simulink model "Now_create_a_Simulink_subsystem_which_takes_ut"  (R2021a)
settings: Solver=VariableStepAuto  StartTime=0.0  StopTime=10.0  RelTol=1e-3
libraries: dsparch4 x2, dspsigops x2, commsynccomp2 x2, simulink x2
settings Model: Creator=Fatiha  LastModifiedBy=Fatiha

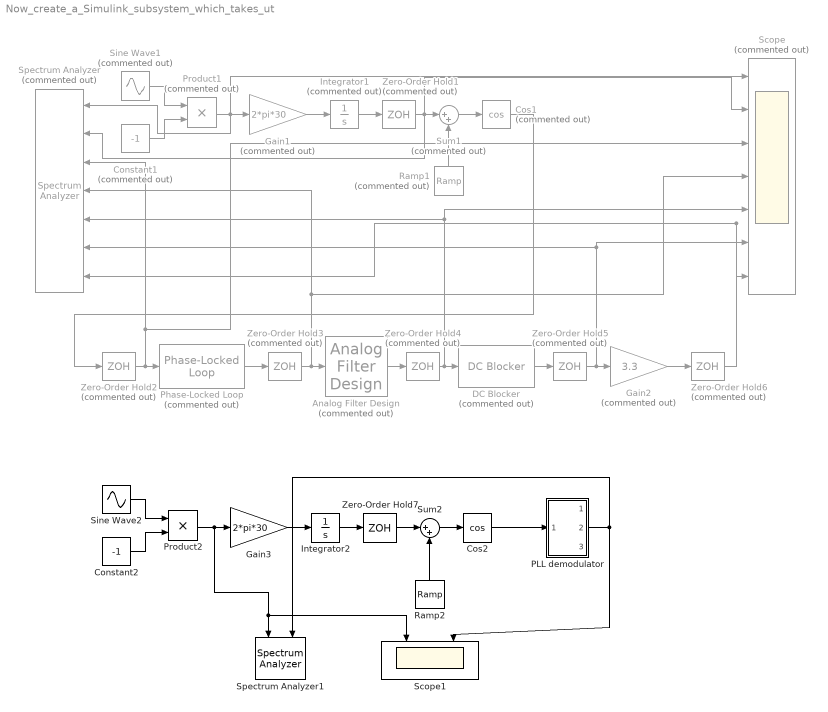
== system Now_create_a_Simulink_subsystem_which_takes_ut ==
  Analog Filter Design : dsparch4/Analog Filter Design  Commented=on  method=Butterworth  filttype=Lowpass  N=8  Wlo=2*pi*200  Whi=80  Rp=2  Rs=40
  Constant1 : Constant  Commented=on  Value=-1  SampleTime=0.00001
  Constant2 : Constant  Value=-1  SampleTime=0.00001
  Cos1 : Trigonometry  Commented=on  Operator=cos  OutputSignalType=real
  Cos2 : Trigonometry  Operator=cos  OutputSignalType=real
  DC Blocker : dspsigops/DC Blocker  Commented=on  Algorithm=IIR  NormalizedBandwidth=0.001  Length=8  Order=6  SimulateUsing=Code generation
      settings: SourceProductBaseCode=DS
  Gain1 : Gain  Commented=on  Gain=2*pi*30
  Gain2 : Gain  Commented=on  Gain=3.3
  Gain3 : Gain  Gain=2*pi*30
  Integrator1 : Integrator  Commented=on
  Integrator2 : Integrator
  PLL demodulator : Subsystem
  Phase-Locked Loop : commsynccomp2/Phase-Locked Loop  Commented=on  Fn="[3.0002  0  40002]"  Fd="[1   67.46   2270.9   40002]"  Kvco=1  Fc=200  Ph=0  Ac=1
      settings: SourceProductBaseCode=CM
  Product1 : Product  Commented=on
  Product2 : Product
  Ramp1 : simulink/Sources/Ramp  Commented=on  slope=2*pi*200  start=0  InitialOutput=0
  Ramp2 : simulink/Sources/Ramp  slope=2*pi*200  start=0  InitialOutput=0
  Scope : Scope  Commented=on  NumInputPorts=7
  Scope1 : Scope  NumInputPorts=2
  Sine Wave1 : Sin  Commented=on  Frequency=2*pi*50  SampleTime=0.00001
  Sine Wave2 : Sin  Frequency=2*pi*50  SampleTime=0.00001
  Spectrum Analyzer : SpectrumAnalyzer  Commented=on  NumInputPorts=7
  Spectrum Analyzer1 : SpectrumAnalyzer  NumInputPorts=2
  Sum1 : Sum  Commented=on  Inputs=|++
  Sum2 : Sum  Inputs=|++
  Zero-Order Hold{1..6} (6 alike) : ZeroOrderHold  Commented=on  SampleTime=0.00001
  Zero-Order Hold7 : ZeroOrderHold  SampleTime=0.00001
  wires:
  Gain1/1 -> Integrator1/1
  Sine Wave1/1 -> Product1/1
  Sum1/1 -> Cos1/1
  Constant1/1 -> Product1/2
  Product1/1 -> Spectrum Analyzer/1, Scope/1, Gain1/1
  Ramp1/1 -> Sum1/2
  Zero-Order Hold4/1 -> Spectrum Analyzer/5, Scope/5, DC Blocker/1
  Integrator1/1 -> Zero-Order Hold1/1
  Zero-Order Hold1/1 -> Spectrum Analyzer/2, Scope/2, Sum1/1
  Cos1/1 -> Zero-Order Hold2/1
  Zero-Order Hold2/1 -> Spectrum Analyzer/3, Scope/3, Phase-Locked Loop/1
  Phase-Locked Loop/2 -> Zero-Order Hold3/1
  Zero-Order Hold3/1 -> Spectrum Analyzer/4, Scope/4, Analog Filter Design/1
  Analog Filter Design/1 -> Zero-Order Hold4/1
  DC Blocker/1 -> Zero-Order Hold5/1
  Zero-Order Hold5/1 -> Scope/6, Spectrum Analyzer/6, Gain2/1
  Gain2/1 -> Zero-Order Hold6/1
  Zero-Order Hold6/1 -> Scope/7, Spectrum Analyzer/7
  Ramp2/1 -> Sum2/2
  Zero-Order Hold7/1 -> Sum2/1
  Integrator2/1 -> Zero-Order Hold7/1
  Product2/1 -> Scope1/1, Spectrum Analyzer1/1, Gain3/1
  Sum2/1 -> Cos2/1
  Constant2/1 -> Product2/2
  Gain3/1 -> Integrator2/1
  Sine Wave2/1 -> Product2/1
  Cos2/1 -> PLL demodulator/1(In1)
  PLL demodulator/2(Out2) -> Scope1/2, Spectrum Analyzer1/2

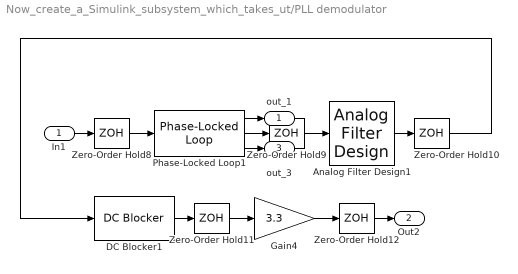
== system Now_create_a_Simulink_subsystem_which_takes_ut/PLL demodulator ==
  In1 : Inport
  Analog Filter Design1 : dsparch4/Analog Filter Design  method=Butterworth  filttype=Lowpass  N=8  Wlo=2*pi*200  Whi=80  Rp=2  Rs=40
  DC Blocker1 : dspsigops/DC Blocker  Algorithm=IIR  NormalizedBandwidth=0.001  Length=8  Order=6  SimulateUsing=Code generation
      settings: SourceProductBaseCode=DS
  Gain4 : Gain  Gain=3.3
  Phase-Locked Loop1 : commsynccomp2/Phase-Locked Loop  Fn="[3.0002  0  40002]"  Fd="[1   67.46   2270.9   40002]"  Kvco=1  Fc=200  Ph=0  Ac=1
      settings: SourceProductBaseCode=CM
  Zero-Order Hold{8..12} (5 alike) : ZeroOrderHold  SampleTime=0.00001
  out_1 : Outport
  Out2 : Outport  Port=2
  out_3 : Outport  Port=3
  wires:
  Phase-Locked Loop1/2 -> Zero-Order Hold9/1
  Zero-Order Hold11/1 -> Gain4/1
  Gain4/1 -> Zero-Order Hold12/1
  Analog Filter Design1/1 -> Zero-Order Hold10/1
  Zero-Order Hold10/1 -> DC Blocker1/1
  DC Blocker1/1 -> Zero-Order Hold11/1
  Zero-Order Hold9/1 -> Analog Filter Design1/1
  Zero-Order Hold8/1 -> Phase-Locked Loop1/1
  Phase-Locked Loop1/3 -> out_3/1
  Phase-Locked Loop1/1 -> out_1/1
  In1/1 -> Zero-Order Hold8/1
  Zero-Order Hold12/1 -> Out2/1
